simulink model "lineal"  (R2022a)
settings: Solver=VariableStepAuto  StartTime=0.0  StopTime=inf  RelTol=1e-3
undefined symbols (not defined in the file or in its folder): gray, none, Rec, SDTV, videoinput
libraries: visionstatistics x2, visionconversions x2, imaqlib x1
settings Model: Creator=misog  LastModifiedBy=misog

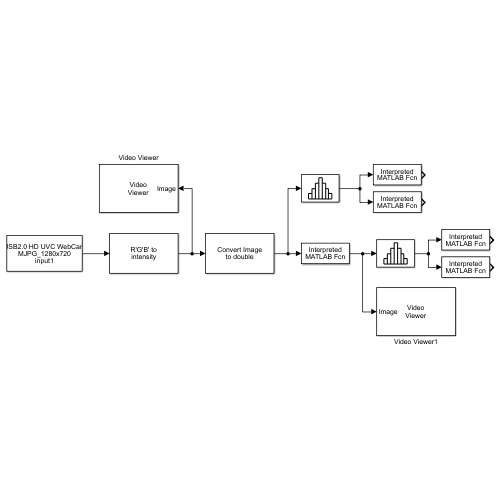
[thumbnail: Simulink's stored preview of the top-level diagram]
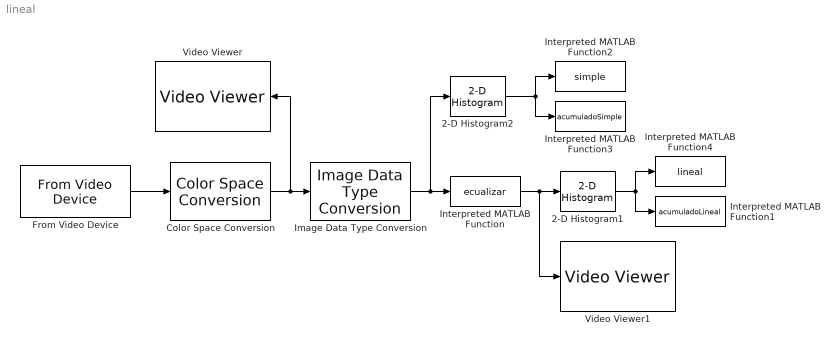
== system lineal ==
  2-D Histogram1 : visionstatistics/2-D Histogram  umin=0  umax=1  nbins=256  operateOver=Entire input  normalized=on  run=off  reset=on  trigtype=None  Dimension=1  colComp=on  roundingMode=Floor  overflowMode=off
      settings: SourceProductBaseCode=VP
  2-D Histogram2 : visionstatistics/2-D Histogram  umin=0  umax=1  nbins=256  operateOver=Entire input  normalized=on  run=off  reset=on  trigtype=None  Dimension=1  colComp=on  roundingMode=Floor  overflowMode=off
      settings: SourceProductBaseCode=VP
  Color Space Conversion : visionconversions/Color Space  Conversion  conversion=Obsolete  conversionActive=R'G'B' to intensity  wp_str=D65  rec=Rec. 601 (SDTV)  sys=1125/60/2:1  imagePorts=One multidimensional signal
  From Video Device : imaqlib/From Video Device  DeviceMenu=winvideo 1 (USB2.0 HD UVC WebCam)  Device=winvideo 1 (USB2.0 HD UVC WebCam)  ObjConstructor=videoinput('winvideo', 1)  VideoFormatMenu=MJPG_1280x720  VideoFormat=MJPG_1280x720  VideoSource=input1  ROIPosition=[0 0 720 1280]  EnableHWTrigger=off  TriggerConfiguration=none/none  SampleTime=1/30  OutputPortsMode=One multidimensional signal  DataType=single  CanDoHWTrigger=no  ReturnedColorSpace=rgb  BlockHandle=4.0002  ROIWidth=1280  ROIHeight=720  ROIColumn=0  ROIRow=0  EngXMLPath=C:\Program Files\MATLAB\R2022a\toolbox\imaq\imaq\private  DevXMLPath=C:\ProgramData\MATLAB\SupportPackages\R2022a\toolbox\imaq\supportpackages\genericvideo\adaptor\win64  EngLibPath=C:\Program Files\MATLAB\R2022a\toolbox\imaq\imaqblks\imaqmex\win64  ColorSpace=rgb  BayerSensorAlignment=grbg  ImaqMode=off
  Image Data Type Conversion : visionconversions/Image Data Type Conversion  outDT=double  isSigned=on  wordLen=16  numFracBits=0
      settings: SourceProductBaseCode=VP
  Interpreted MATLAB Function : MATLABFcn  MATLABFcn=ecualizar  Output1D=off
  Interpreted MATLAB Function1 : MATLABFcn  MATLABFcn=acumuladoLineal  Output1D=off
  Interpreted MATLAB Function2 : MATLABFcn  MATLABFcn=simple  Output1D=off
  Interpreted MATLAB Function3 : MATLABFcn  MATLABFcn=acumuladoSimple  Output1D=off
  Interpreted MATLAB Function4 : MATLABFcn  MATLABFcn=lineal  Output1D=off
  Video Viewer : VideoViewer  colormapValue=gray(256)  FigPos=[962 513 958 405]
  Video Viewer1 : VideoViewer  colormapValue=gray(256)  FigPos=[962 1029 958 405]
  wires:
  From Video Device/1 -> Color Space Conversion/1
  Color Space Conversion/1 -> Image Data Type Conversion/1, Video Viewer/1
  Image Data Type Conversion/1 -> 2-D Histogram2/1, Interpreted MATLAB Function/1
  Interpreted MATLAB Function/1 -> Video Viewer1/1, 2-D Histogram1/1
  2-D Histogram1/1 -> Interpreted MATLAB Function4/1, Interpreted MATLAB Function1/1
  2-D Histogram2/1 -> Interpreted MATLAB Function3/1, Interpreted MATLAB Function2/1
